simulink library "moving_average_filter_cc"  (R2025b)
settings: Solver=VariableStepAuto  StartTime=0.0  StopTime=10.0  RelTol=1e-3
undefined symbols (not defined in the file): ts_afe
libraries: simulink x1
settings Model: Creator=dbagn  LastModifiedBy=dbagn
settings SFSimCC: SimCustomHeaderCode=|
  | #include "dsmavgflt.h"
  | #include "dsmavgflt_simulink.h"
  | #include "mavgflt.h"
  | #include "mavgflt_simulink.h"
  | #include "mavgflts.h"
  | #include "mavgflts_simulink.h"
settings SFSimCC: SimUserSources=|
  | "dsmavgflt_simulink.c"
  | "dsmavgflt.c"
  | "mavgflts_simulink.c"
  | "mavgflts.c"
  | "mavgflt_simulink.c"
  | "mavgflt.c"
settings SFSimCC: SimUserIncludeDirs=|
  | include
  | src

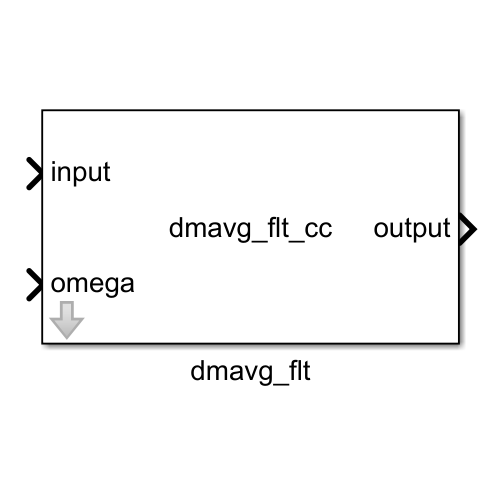
[thumbnail: Simulink's stored preview of the top-level diagram]
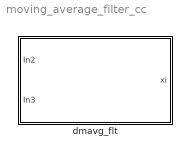
== system moving_average_filter_cc ==
  dmavg_flt : Subsystem  mask{instance=0, ts=ts_afe, enable_time=0.025}
      mask prompts: ts "sampling time (s)"; enable_time "enable_time (s)"
      mask Display:
      | disp('dmavg_flt_cc');
      | port_label('input', 1, 'input');
      | port_label('input', 2, 'omega');
      | port_label('output', 1, 'output');

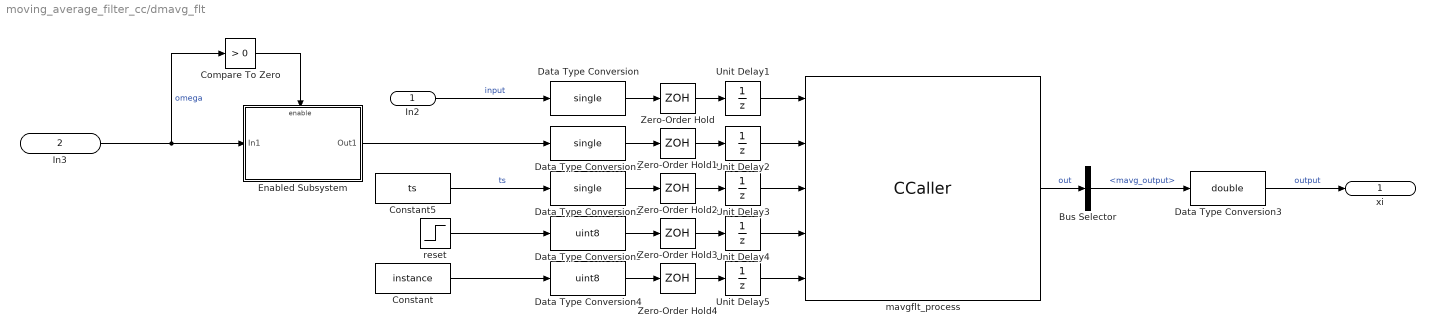
== system moving_average_filter_cc/dmavg_flt ==
  In2 : Inport
  In3 : Inport  Port=2
  Bus Selector : BusSelector  OutputSignals=mavg_output
  Compare To Zero : simulink/Logic and Bit Operations/Compare To Zero  relop=>  OutDataTypeStr=boolean
  Constant : Constant  Value=instance
  Constant5 : Constant  Value=ts
  Data Type Conversion : DataTypeConversion  OutDataTypeStr=single  SaturateOnIntegerOverflow=off  RndMeth=Floor
  Data Type Conversion1 : DataTypeConversion  OutDataTypeStr=single  SaturateOnIntegerOverflow=off  RndMeth=Floor
  Data Type Conversion2 : DataTypeConversion  OutDataTypeStr=single  SaturateOnIntegerOverflow=off  RndMeth=Floor
  Data Type Conversion3 : DataTypeConversion  OutDataTypeStr=double  SaturateOnIntegerOverflow=off  RndMeth=Floor
  Data Type Conversion4 : DataTypeConversion  OutDataTypeStr=uint8  SaturateOnIntegerOverflow=off  RndMeth=Floor
  Data Type Conversion5 : DataTypeConversion  OutDataTypeStr=uint8  SaturateOnIntegerOverflow=off  RndMeth=Floor
  Enabled Subsystem : Subsystem  TreatAsAtomicUnit=on
  Unit Delay{1..5} (5 alike) : UnitDelay  SampleTime=-1  HasFrameUpgradeWarning=on
  Zero-Order Hold{,1..4} (5 alike) : ZeroOrderHold  SampleTime=-1
  mavgflt_process : CCaller  FunctionName=mavgflt_process_simulink  PortSpecificationStruct="%)30     .    B H   8    (     @         %    \"     8    !     0         %  0 \"0    $    _    07)G3F%M90  4&]R=$YA;64 4V-O<&4     26YD97@     5'EP90      4VEZ90      27-';&]B86P   X    P    !@    @    $          4    (     0    ,    !         !   P!O=70 #@   #     &    \"     0         !0    @    !     P    $         $  # &]U=  .    .     8    (    !          %    \"     $    &     0         0   ...(+3251 chars)"
  reset : Step  Time=enable_time  Before=1  After=0
  xi : Outport
  wires:
  Bus Selector/1 -> Data Type Conversion3/1  "<mavg_output>"
  mavgflt_process/1 -> Bus Selector/1  "out"
  Zero-Order Hold4/1 -> Unit Delay5/1
  Zero-Order Hold3/1 -> Unit Delay4/1
  Zero-Order Hold2/1 -> Unit Delay3/1
  Zero-Order Hold1/1 -> Unit Delay2/1
  Zero-Order Hold/1 -> Unit Delay1/1
  Unit Delay5/1 -> mavgflt_process/5
  Unit Delay4/1 -> mavgflt_process/4
  Unit Delay3/1 -> mavgflt_process/3
  Unit Delay2/1 -> mavgflt_process/2
  Unit Delay1/1 -> mavgflt_process/1
  Data Type Conversion3/1 -> xi/1  "output"
  Enabled Subsystem/1(Out1) -> Data Type Conversion1/1
  Compare To Zero/1 -> Enabled Subsystem/Enable
  In3/1 -> Enabled Subsystem/1(In1), Compare To Zero/1  "omega"
  Constant5/1 -> Data Type Conversion2/1  "ts"
  In2/1 -> Data Type Conversion/1  "input"
  reset/1 -> Data Type Conversion5/1
  Constant/1 -> Data Type Conversion4/1
  Data Type Conversion/1 -> Zero-Order Hold/1
  Data Type Conversion1/1 -> Zero-Order Hold1/1
  Data Type Conversion2/1 -> Zero-Order Hold2/1
  Data Type Conversion5/1 -> Zero-Order Hold3/1
  Data Type Conversion4/1 -> Zero-Order Hold4/1

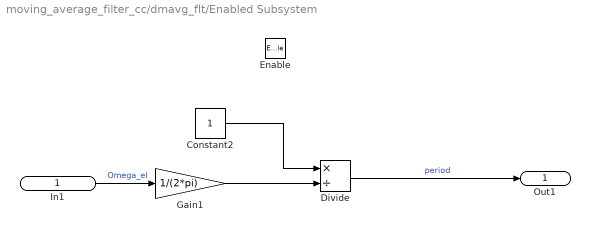
== system moving_average_filter_cc/dmavg_flt/Enabled Subsystem ==
  In1 : Inport
  Enable : EnablePort
  Constant2 : Constant
  Divide : Product  Inputs=*/
  Gain1 : Gain  Gain=1/(2*pi)
  Out1 : Outport
  wires:
  Divide/1 -> Out1/1  "period"
  Gain1/1 -> Divide/2
  In1/1 -> Gain1/1  "Omega_el"
  Constant2/1 -> Divide/1
